simulink library "QuadModelLib1"  (R2022a)
settings: Solver=VariableStepAuto  StartTime=0.0  StopTime=10.0  RelTol=1e-3
values from neighbouring files (symbols this model uses):
  ModelParam_envAltitude = -50    [Init.m]
  ModelParam_noisePowerIMU = 0    [Init.m]
  ModelParam_timeSampBaro = 0.01    [Init.m]
  MotorFault1 = MotorFaultTemp    [Init.m]
undefined symbols (not defined in the file or in its folder): BatteryFault, Earth, F, FaultParamAPI, Light, LoadFault, MIL, ModelParam_noiseLowPassFilterCoeAccel, ModelParam_noiseLowPassFilterCoeGyro, Moderate, PropFault, SensorFault, WGS84, WindFault
libraries: aerolibwind2 x4, aerolibtransform2 x1, simulink x1, aerolibasang x1, aerolibatmos2 x1, aerolibnav x1, aerolibgravity2 x1
(part 2 of 2)

== matlab function QuadModelLib1/SensorFault/baro NoiseFun ==
  settings: updateMethod=DISCRETE
  data: BaroIn input; isBaroFault input; y output; BaroFaultParams input
function y = BaroFaultFun(BaroIn,isBaroFault,BaroFaultParams)
    y = BaroIn;
    
    if isBaroFault
        flag = BaroFaultParams(1);
        
       
        if flag == 1
            y = BaroFaultParams(2);
        elseif flag == 2
            y = y + BaroFaultParams(2);
        elseif flag == 3
            mean = BaroFaultParams(2);
            stddev = BaroFaultParams(3);
            y = y + generate_wgn(mean,stddev);
        elseif flag == 4
            y = y * BaroFaultParams(2);
        end

    end

end

function y = generate_wgn(mean,stddev)
    persistent V1 V2 S phase

    if isempty(phase)
        phase = true;
        V1 = 0; 
        V2 = 0; 
        S = 0; 
    end
    
    if phase
        while true
            U1 = rand();
            U2 = rand();
            V1 = 2.0 * U1 - 1.0;
            V2 = 2.0 * U2 - 1.0;
            S = V1 * V1 + V2 * V2;
            if S < 1.0 && abs(S) >= 1e-8
                break;
            end
        end
        X = V1 * sqrt(-2.0 * log(S) / S);
    else
        X = V2 * sqrt(-2.0 * log(S) / S);
    end
    
    y = mean + stddev * X;
  
    phase = ~phase;

end

== matlab function QuadModelLib1/GPSFault/Acc NoiseFun ==
  settings: updateMethod=DISCRETE
  data: GPSIn input; y output; isGPSFault input; GPSFaultParams input; satellites output; GPS3Dfixed output
function [y, satellites, GPS3Dfixed] = GPSFaultFun(GPSIn,isGPSFault,GPSFaultParams)
    y = GPSIn;
    satellites = 10;
    GPS3Dfixed = 3;
    
    if isGPSFault
        % FaultParams(1)为标志位
        flag = GPSFaultParams(1);
        
        % 覆盖模式，当为-1时，保持原有输出
        if flag == 1
            for ind = 1:3
                if GPSFaultParams(ind+1) ~= -1
                    y(ind) = GPSFaultParams(ind+1);
                end
            end
        
        % 叠加模式，当为-1时，保持原有输出
        elseif flag == 2
            for ind = 1:3
                if GPSFaultParams(ind+1) ~= -1
                    y(ind) = y(ind) + GPSFaultParams(ind+1);
                end
            end

        % 噪声模式，当为-1时，保持原有输出
        elseif flag == 3
            mean = GPSFaultParams(2);
            stddev = GPSFaultParams(3);
            for ind = 1:3
                if GPSFaultParams(ind+3) ~= -1
                    y(ind) = y(ind) + generate_wgn(mean,stddev);
                end
            end

        % 尺度因子模式，当为-1时，保持原有输出
        elseif flag == 4
            for ind = 1:3
                if GPSFaultParams(ind+1) ~= -1
                    y(ind) = y(ind) * GPSFaultParams(ind+1);
                end
            end

        % 改变搜星数
        elseif flag == 5
           satellites = GPSFaultParams(2);

        % 改变Fixed
        elseif flag == 6
           GPS3Dfixed = GPSFaultParams(2);
           
        end
        

    end

end

function y = generate_wgn(mean,stddev)
    persistent V1 V2 S phase

    if isempty(phase)
        phase = true;
        V1 = 0;
        V2 = 0;
        S = 0;
    end
    
    if phase
        while true
            U1 = rand();
            U2 = rand();
            V1 = 2.0 * U1 - 1.0;
            V2 = 2.0 * U2 - 1.0;
            S = V1 * V1 + V2 * V2;
            if S < 1.0 && abs(S) >= 1e-8
                break;
            end
        end
        X = V1 * sqrt(-2.0 * log(S) / S);
    else
        X = V2 * sqrt(-2.0 * log(S) / S);
    end
    
    y = mean + stddev * X;
  
    phase = ~phase;

end

== matlab function QuadModelLib1/SensorFault/FaultParamsExtract1 ==
  settings: updateMethod=DISCRETE
  data: FaultID input; inInts input; hasFault_gyro output; inFloats input; FaultParam output
function [hasFault_gyro, FaultParam] = fcn(FaultID,inInts,inFloats)
persistent hFault;
persistent fParam;

if isempty(hFault)
    hFault=false;
end
if isempty(fParam)
    fParam=zeros(20,1);
end

hFaultTmp=false;
fParamTmp=zeros(20,1);
j=1;
for i=1:8
    if inInts(i) == FaultID
        hFaultTmp=true;
        fParamTmp(2*j-1)=inFloats(2*i-1);
        fParamTmp(2*j)=inFloats(2*i);
        j=j+1;
    end
end
if hFaultTmp
    hFault=hFaultTmp;
    fParamTmp(17:20) = inFloats(17:20);
    fParam=fParamTmp;
end

hasFault_gyro=hFault;
FaultParam=fParam;

== matlab function QuadModelLib1/WindFault/MATLAB Function ==
  settings: updateMethod=DISCRETE
  data: t input; isGustWind input; gWind output; GustWindParams input; turb input
function gWind = GustWindModel(t,isGustWind,GustWindParams,turb)

if(GustWindParams(2)<1)
    GustWindParams(2)=1;
end
timeVel=60/GustWindParams(2);

vmax=GustWindParams(1);

persistent t0;
if isempty(t0)
    t0=0;
end

persistent isInGust;
if isempty(isInGust)
    isInGust=0;
end

persistent t1;
if isempty(t1)
    t1=2;
end

persistent a;
if isempty(a)
    a=0.5;
end

persistent ang;
if isempty(ang)
    ang=pi/2;
end

persistent wlast;
if isempty(wlast)
    wlast=vmax*0.5;
end

persistent wNow;
if isempty(wNow)
    wNow=1.4*0.8*vmax;
end


if isGustWind&&isInGust<0.5
    t0=t;
    t1=timeVel*(3/4+1/2*rand(1));
    a=1/4+1/2*rand(1);
    ang=pi*2*rand(1);
    wlast=wNow;
    wNow=1.2*(rand(1)*0.5+0.5)*vmax;
    
    isInGust=1;
end

if ~isGustWind
    isInGust=0;
end

gWind=[0;0;0];

if(t<t0+t1*a)
    gWindMag=(wNow-wlast)/2*(1-cos((t-t0)/(t1*a)*pi))+wlast;
else
    gWindMag=wNow;
end

if abs(t-(t0+t1))<0.05
    rng(t*1000);
    t0=t;
    t1=timeVel*(3/4+1/2*rand(1));
    a=1/4+1/2*rand(1);
    ang=ang+0.1*pi*rand(1);
    wlast=wNow;
    wNow=1.2*(rand(1)*0.5+0.5)*vmax;
end

gWind(1)=gWindMag*cos(ang)*0.8+turb(1)*0.4;
gWind(2)=gWindMag*sin(ang)*0.8+turb(2)*0.4;
gWind(3)=turb(3)*0.4;

== matlab function QuadModelLib1/WindFault/MATLAB Function1 ==
  data: wind output size=3; isConstWind input; isGustWind input; isTurbWind input; isSheerWind input; ConstWind input; GustWind input; TurbWind input; SheerWind input
function wind = WindFun(isConstWind,isGustWind,isTurbWind,isSheerWind,ConstWind,GustWind,TurbWind,SheerWind)
wind=[0;0;0];
if isConstWind
    wind=[ConstWind(1);ConstWind(2);ConstWind(3)];
elseif isGustWind
    wind=GustWind;
elseif isTurbWind
    wind=TurbWind;
elseif isSheerWind
    wind=SheerWind;
end

== matlab function QuadModelLib1/MotorFault/FaultParamsExtract ==
  settings: updateMethod=DISCRETE
  data: FaultID input; inInts input; hasFault output; inFloats input; FaultParam output
function [hasFault, FaultParam] = fcn(FaultID,inInts,inFloats)
persistent hFault;
persistent fParam;

if isempty(hFault)
    hFault=false;
end
if isempty(fParam)
    fParam=zeros(20,1);
end

hFaultTmp=false;
fParamTmp=zeros(20,1);
j=1;

for i=1:8
    if inInts(i) == FaultID
        hFaultTmp=true;
        fParamTmp(2*j-1)=inFloats(2*i-1);
        fParamTmp(2*j)=inFloats(2*i);
        j=j+1;
    end
end
if hFaultTmp
    hFault=hFaultTmp;
    fParamTmp(17:20) = inFloats(17:20);
    fParam=fParamTmp;
end

hasFault=hFault;
FaultParam=fParam;

== matlab function QuadModelLib1/BatteryFault/FaultParamsExtract1 ==
  settings: updateMethod=DISCRETE
  data: FaultID input; inInts input; hasFault_isPowOff output; inFloats input; FaultParam output
function [hasFault_isPowOff, FaultParam] = fcn(FaultID,inInts,inFloats)
persistent hFault;
persistent fParam;

if isempty(hFault)
    hFault=false;
end
if isempty(fParam)
    fParam=zeros(20,1);
end

hFaultTmp=false;
fParamTmp=zeros(20,1);
j=1;
for i=1:8
    if inInts(i) == FaultID
        hFaultTmp=true;
        fParamTmp(2*j-1)=inFloats(2*i-1);
        fParamTmp(2*j)=inFloats(2*i);
        j=j+1;
    end
end
if hFaultTmp
    hFault=hFaultTmp;
    fParamTmp(17:20) = inFloats(17:20);
    fParam=fParamTmp;
end

hasFault_isPowOff=hFault;
FaultParam=fParam;

== matlab function QuadModelLib1/WindFault/FaultParamsExtract1 ==
  settings: updateMethod=DISCRETE
  data: FaultID input; inInts input; hasFault_GustWind output; inFloats input; FaultParam output
function [hasFault_GustWind, FaultParam] = fcn(FaultID,inInts,inFloats)
persistent hFault;
persistent fParam;

if isempty(hFault)
    hFault=false;
end
if isempty(fParam)
    fParam=zeros(20,1);
end

hFaultTmp=false;
fParamTmp=zeros(20,1);
j=1;
for i=1:8
    if inInts(i) == FaultID
        hFaultTmp=true;
        fParamTmp(2*j-1)=inFloats(2*i-1);
        fParamTmp(2*j)=inFloats(2*i);
        j=j+1;
    end
end
if hFaultTmp
    hFault=hFaultTmp;
    fParamTmp(17:20) = inFloats(17:20);
    fParam=fParamTmp;
end

hasFault_GustWind=hFault;
FaultParam=fParam;

== matlab function QuadModelLib1/WindFault/FaultParamsExtract4 ==
  settings: updateMethod=DISCRETE
  data: FaultID input; inInts input; hasFault_WindNoise output; inFloats input; FaultParam output
function [hasFault_WindNoise, FaultParam] = fcn(FaultID,inInts,inFloats)
persistent hFault;
persistent fParam;

if isempty(hFault)
    hFault=false;
end
if isempty(fParam)
    fParam=zeros(20,1);
end

hFaultTmp=false;
fParamTmp=zeros(20,1);
j=1;
for i=1:8
    if inInts(i) == FaultID
        hFaultTmp=true;
        fParamTmp(2*j-1)=inFloats(2*i-1);
        fParamTmp(2*j)=inFloats(2*i);
        j=j+1;
    end
end
if hFaultTmp
    hFault=hFaultTmp;
    fParamTmp(17:20) = inFloats(17:20);
    fParam=fParamTmp;
end

hasFault_WindNoise=hFault;
FaultParam=fParam;
